simulink model "lev"  (R2021b)
settings: Solver=ode3  StartTime=0.0  StopTime=35  FixedStep=1e-4  RelTol=1e-3
values from neighbouring files (symbols this model uses):
  g = s(1:n,n+1:n+nb)    [MagLev.m]    (also in MagLev4coils.m = 9.8)
  K = m*g*x1*x1/i/i    (= 0.00013716864)    [MagLev.m]    (also in MagLev4coils.m = m*g*z1*z1/i/i)
  L = 0.00392    [MagLev.m]    (also in MagLev4coils.m = 0.00388)
  m = 0.03    [MagLev.m]    (also in MagLev4coils.m = 0.01)
  R = 10.8    [MagLev.m]    (also in MagLev4coils.m = 4)
settings Model: Creator=ik76  LastModifiedBy=ik76
settings SolverCC: ZeroCrossAlgorithm=Adaptive
settings OptimizationCC: BlockReduction=off  BooleanDataType=off
settings DebuggingCC: SaveWithParameterizedLinksMsg=none  UnderspecifiedInitializationDetection=Classic  MergeDetectMultiDrivingBlocksExec=none  SignalResolutionControl=TryResolveAllWithWarning  IgnoredZcDiagnostic=none
settings HardwareCC: TargetUnknown=on
settings ModelReferenceCC: PropagateSignalLabelsOutOfModel=off

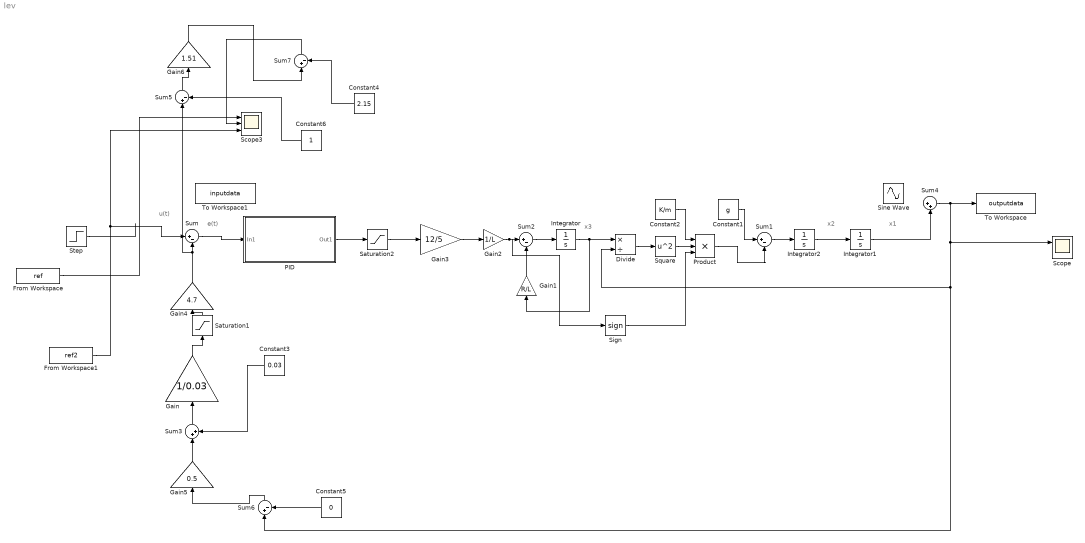
== system lev ==
  note: x3
  note: x2
  note: x1
  note: e(t)
  note: u(t)
  Constant1 : Constant  Value=g
  Constant2 : Constant  Value=K/m
  Constant3 : Constant  Value=0.03
  Constant4 : Constant  Value=2.15
  Constant5 : Constant  Value=0
  Constant6 : Constant
  Divide : Product  Inputs=*/
  From Workspace : FromWorkspace  VariableName=ref
  From Workspace1 : FromWorkspace  VariableName=ref2
  Gain : Gain  Gain=1/0.03
  Gain1 : Gain  Gain=R/L
  Gain2 : Gain  Gain=1/L
  Gain3 : Gain  Gain=12/5
  Gain4 : Gain  Gain=4.7
  Gain5 : Gain  Gain=0.5
  Gain6 : Gain  Gain=1.51
  Integrator : Integrator
  Integrator1 : Integrator  InitialCondition=-0.015
  Integrator2 : Integrator
  PID : Subsystem
  Product : Product  Inputs=3
  Saturation1 : Saturate  UpperLimit=1  LowerLimit=0
  Saturation2 : Saturate  UpperLimit=5  LowerLimit=-5
  Scope : Scope  NumInputPorts=2
  Scope3 : Scope  NumInputPorts=3
  Sign : Signum
  Sine Wave : Sin  Amplitude=-0.005  Frequency=200  SampleTime=0
  Square : Math  Operator=square  SaturateOnIntegerOverflow=on
  Step : Step  Time=0  After=2.5  SampleTime=0
  Sum{,1..2,5..7} (6 alike) : Sum  Inputs=|+-
  Sum3 : Sum  Inputs=|++
  Sum4 : Sum  Inputs=|++
  To Workspace : ToWorkspace  VariableName=outputdata  SaveFormat=Structure With Time  SampleTime=-1
  To Workspace1 : ToWorkspace  VariableName=inputdata  SaveFormat=Structure With Time  SampleTime=-1
  wires:
  Gain2/1 -> Sign/1, Sum2/1
  Gain1/1 -> Sum2/2
  Sum2/1 -> Integrator/1
  Integrator/1 -> Divide/1, Gain1/1
  Divide/1 -> Square/1
  Square/1 -> Product/2
  Product/1 -> Sum1/2
  Sum1/1 -> Integrator2/1
  Constant2/1 -> Product/1
  Saturation1/1 -> Gain4/1
  Integrator2/1 -> Integrator1/1
  Constant1/1 -> Sum1/1
  Sign/1 -> Product/3
  Gain/1 -> Saturation1/1
  Sum3/1 -> Gain/1
  Constant3/1 -> Sum3/2
  Sum/1 -> PID/1(In1)
  Gain3/1 -> Gain2/1
  Sum4/1 -> Sum6/1, Divide/2, Scope/1, To Workspace/1
  PID/1(Out1) -> Saturation2/1
  From Workspace1/1 -> Sum/1, Scope3/3
  Step/1 -> ?
  Saturation2/1 -> Gain3/1
  From Workspace/1 -> Scope3/1
  Integrator1/1 -> Sum4/2
  Gain4/1 -> Sum5/1, Sum/2
  Gain5/1 -> Sum3/1
  Constant5/1 -> Sum6/2
  Sum6/1 -> Gain5/1
  Constant4/1 -> Sum7/2
  Sum5/1 -> Gain6/1
  Gain6/1 -> Sum7/1
  Sum7/1 -> Scope3/2
  Constant6/1 -> Sum5/2

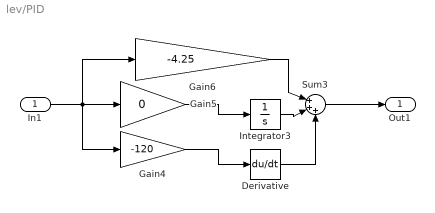
== system lev/PID ==
  In1 : Inport
  Derivative : Derivative
  Gain4 : Gain  Gain=-120
  Gain5 : Gain  Gain=0
  Gain6 : Gain  Gain=-4.25
  Integrator3 : Integrator
  Sum3 : Sum  Inputs=|+++
  Out1 : Outport
  wires:
  Gain6/1 -> Sum3/1
  In1/1 -> Gain4/1, Gain6/1, Gain5/1
  Gain5/1 -> Integrator3/1
  Integrator3/1 -> Sum3/2
  Gain4/1 -> Derivative/1
  Derivative/1 -> Sum3/3
  Sum3/1 -> Out1/1
